simulink model "ball_sim"  (R2018a)
settings: Solver=ode45  StartTime=0.0  StopTime=1000  RelTol=1e-3  EnableMultiTasking=on
InitFcn:
  | param
undefined symbols (not defined in the file or in its folder): ball_ctrl, draw_ball_beam, P
libraries: simulink x1
settings Model: Creator=beard  LastModifiedBy=mouse
settings DataIOCC: LimitDataPoints=on  SaveFormat=Array  SignalLoggingSaveFormat=ModelDataLogs
settings OptimizationCC: ExpressionDepthLimit=2147483647  InitFltsAndDblsToZero=on  LifeSpan=inf
settings DebuggingCC: UnderspecifiedInitializationDetection=Classic  MergeDetectMultiDrivingBlocksExec=none  SolverPrmCheckMsg=warning  FcnCallInpInsideContextMsg=warning  StateNameClashWarn=warning  SFUnexpectedBacktrackingDiag=warning  SFNoUnconditionalDefaultTransitionDiag=warning  SFExecutionAtInitializationDiag=none
settings HardwareCC: ProdBitPerPointer=32  ProdBitPerSizeT=32  ProdBitPerPtrDiffT=32  ProdLargestAtomicFloat=None  ProdIntDivRoundTo=Undefined  ProdEndianess=Unspecified  ProdWordSize=32  ProdHWDeviceType=32-bit Generic
settings ModelReferenceCC: PropagateSignalLabelsOutOfModel=off
settings CodeAppCC: StateflowObjectComments=on
settings GRTTargetCC: TargetLangStandard=C89/C90 (ANSI)  GeneratePreprocessorConditionals=Disable all  CombineOutputUpdateFcns=off  GRTInterface=on
settings ConfigComp: CovMetricSettings=dw  CovHtmlReporting=on  CovSaveCumulativeToWorkspaceVar=on  CovSaveSingleToWorkspaceVar=on  CovExternalEMLEnable=off

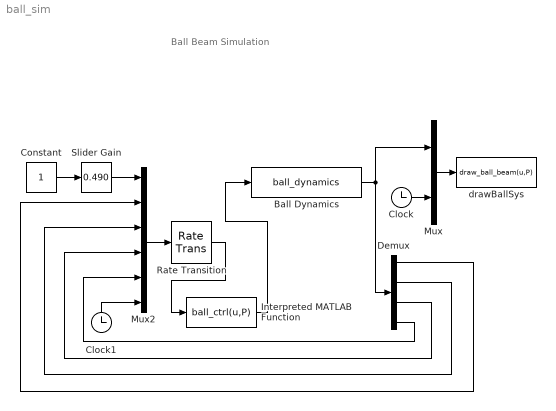
== system ball_sim ==
  note: Ball Beam Simulation
  Ball Dynamics : S-Function  FunctionName=ball_dynamics  Parameters=P  SFunctionDeploymentMode=off  EnableBusSupport=off
  Clock : Clock
  Clock1 : Clock
  Constant : Constant
  Demux : Demux
  Interpreted MATLAB Function : MATLABFcn  MATLABFcn=ball_ctrl(u,P)  OutputDimensions=1
  Mux : Mux  Inputs=2
  Mux2 : Mux  Inputs=6
  Rate Transition : RateTransition  OutPortSampleTime=P.Ts
  Slider Gain : simulink/Math Operations/Slider Gain  gain=0.490  low=0  high=.5
  drawBallSys : MATLABFcn  MATLABFcn=draw_ball_beam(u,P)  OutputDimensions=0  SampleTime=.5
  wires:
  Mux/1 -> drawBallSys/1
  Clock/1 -> Mux/2
  Ball Dynamics/1 -> Mux/1, Demux/1
  Slider Gain/1 -> Mux2/1
  Mux2/1 -> Rate Transition/1
  Demux/1 -> Mux2/2
  Demux/2 -> Mux2/3
  Clock1/1 -> Mux2/6
  Rate Transition/1 -> Interpreted MATLAB Function/1
  Interpreted MATLAB Function/1 -> Ball Dynamics/1
  Demux/4 -> Mux2/5
  Demux/3 -> Mux2/4
  Constant/1 -> Slider Gain/1
